simulink model "task5"  (R2022b)
settings: Solver=FixedStepAuto  StartTime=0.0  StopTime=7  RelTol=1e-8
undefined symbols (not defined in the file): ki, kp
settings Model: Creator=anton  LastModifiedBy=anton
settings DataIOCC: ExternalInput=data  LoadExternalInput=on

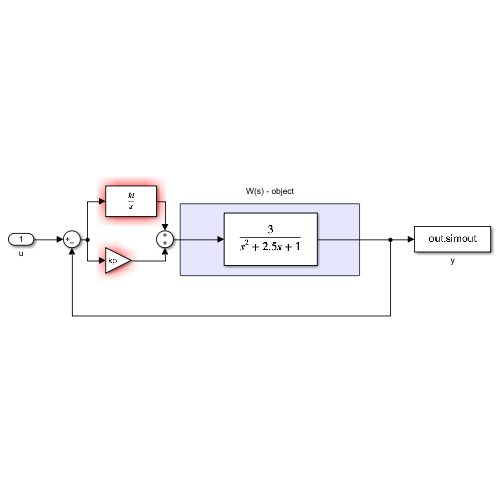
[thumbnail: Simulink's stored preview of the top-level diagram]
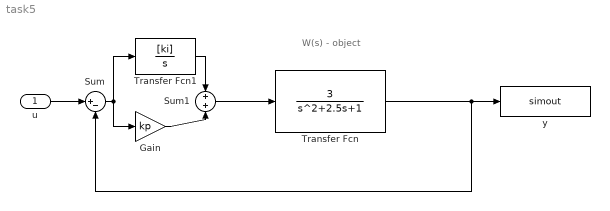
== system task5 ==
  note: W(s) - object
  u : Inport
  Gain : Gain  Gain=kp
  Sum : Sum  Inputs=|+-
  Sum1 : Sum
  Transfer Fcn : TransferFcn  Numerator=[3]  Denominator=[1 2.5 1]
  Transfer Fcn1 : TransferFcn  Numerator=[ki]  Denominator=[1 0]
  y : ToWorkspace  VariableName=simout  SaveFormat=Timeseries  SampleTime=-1
  wires:
  u/1 -> Sum/1
  Sum/1 -> Gain/1, Transfer Fcn1/1
  Transfer Fcn/1 -> Sum/2, y/1
  Sum1/1 -> Transfer Fcn/1
  Gain/1 -> Sum1/2
  Transfer Fcn1/1 -> Sum1/1
